simulink subsystem "InverseServoValveLinkage"  (R2020b)
settings: Solver=VariableStepAuto  StartTime=0.0  StopTime=10.0  RelTol=1e-3
model mask{servoValveSignConvention=ServoValveSignConvention.POSITIVE_AWAY_FROM_VALVE, valveCloseHandleRotationDirection=ValveCloseHandleRotationDirection.AWAY_FROM_SERVO, g=21, a=10.17, h=30.625, b=20.78, linkageServoAngleForClosedDegrees=217, servoCommandedCloseAngleDegrees=0}
  mask prompts: servoValveSignConvention "Servo valve sign convention"; valveCloseHandleRotationDirection "Valve handle close direction"; g "Distance between pivots (mm)"; a "Length of crank arm (mm)"; h "Length of coupler arm (mm)"; b "Length of rocket arm (mm)"; linkageServoAngleForClosedDegrees "Servo angle for closed valve degrees (in linkage angle convention)"; servoCommandedCloseAngleDegrees "Angle to command to servo for closed valve degrees"
undefined symbols (not defined in the file or in its folder): linkageValveAngleForOpenDegrees
settings Model: Creator=Edward  LastModifiedBy=Edward

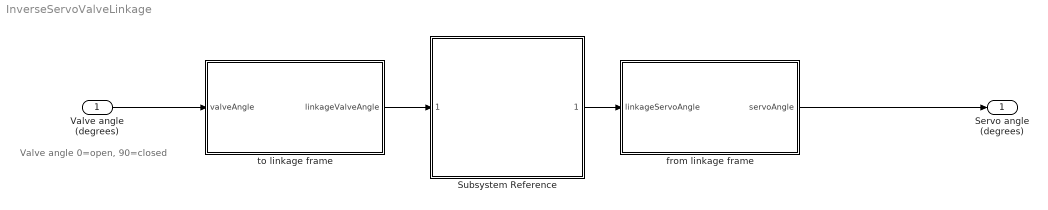
== system InverseServoValveLinkage ==
  note: Valve angle 0=open, 90=closed
  Valve angle (degrees) : Inport
  Subsystem Reference : Subsystem  ReferencedSubsystem=AnalyticInverseFourBarLinkage  g=g  a=a  h=h  b=b  solutionSelector=1
  from linkage frame : MATLAB Function  TreatAsAtomicUnit=on
  to linkage frame : MATLAB Function  TreatAsAtomicUnit=on
  Servo angle (degrees) : Outport
  wires:
  from linkage frame/1(servoAngle) -> Servo angle (degrees)/1
  Valve angle (degrees)/1 -> to linkage frame/1(valveAngle)
  Subsystem Reference/1 -> from linkage frame/1(linkageServoAngle)
  to linkage frame/1(linkageValveAngle) -> Subsystem Reference/1

== matlab function InverseServoValveLinkage/from linkage frame ==
  data: linkageServoAngle input; servoAngle output; linkageServoAngleForClosedDegrees parameter; servoCommandedCloseAngleDegrees parameter; servoValveSignConvention parameter Enum: ServoValveSignConvention; valveCloseHandleRotationDirection parameter Enum: ValveCloseHandleRotationDirection
function servoAngle = fcn(linkageServoAngle, linkageServoAngleForClosedDegrees, ...
servoCommandedCloseAngleDegrees, servoValveSignConvention, valveCloseHandleRotationDirection)
%Get actual servo angle from linkage coordinate system servoAngle
servoAngle = -1;
if(servoValveSignConvention == ServoValveSignConvention.POSITIVE_AWAY_FROM_VALVE)
    if(valveCloseHandleRotationDirection == ValveCloseHandleRotationDirection.TOWARDS_SERVO)
        servoAngle = clampDegreeAngle(linkageServoAngle-linkageServoAngleForClosedDegrees+servoCommandedCloseAngleDegrees);
    elseif(valveCloseHandleRotationDirection == ValveCloseHandleRotationDirection.AWAY_FROM_SERVO)
        servoAngle = clampDegreeAngle(-(linkageServoAngle-linkageServoAngleForClosedDegrees)+servoCommandedCloseAngleDegrees);
    end
elseif (servoValveSignConvention == ServoValveSignConvention.POSITIVE_TOWARDS_VALVE)
    if(valveCloseHandleRotationDirection == ValveCloseHandleRotationDirection.TOWARDS_SERVO)
        servoAngle = clampDegreeAngle(-(linkageServoAngle - servoCommandedCloseAngleDegrees) + linkageServoAngleForClosedDegrees);
    elseif(valveCloseHandleRotationDirection == ValveCloseHandleRotationDirection.AWAY_FROM_SERVO)
        servoAngle = clampDegreeAngle(linkageServoAngle-linkageServoAngleForClosedDegrees+servoCommandedCloseAngleDegrees);
    end
end
if(servoAngle >= 300)
   servoAngle = servoAngle-360; 
end

== matlab function InverseServoValveLinkage/to linkage frame ==
  data: valveAngle input; linkageValveAngle output; linkageValveAngleForOpenDegrees parameter; valveCloseHandleRotationDirection parameter Enum: ValveCloseHandleRotationDirection
function linkageValveAngle = fcn(valveAngle, linkageValveAngleForOpenDegrees, ...
    valveCloseHandleRotationDirection)
%Get actual valve angle (0=open,90=closed) from linkage coordinate system
linkageValveAngle = -1;
if(valveCloseHandleRotationDirection == ValveCloseHandleRotationDirection.TOWARDS_SERVO)
    linkageValveAngle = clampDegreeAngle(valveAngle+linkageValveAngleForOpenDegrees);
elseif(valveCloseHandleRotationDirection == ValveCloseHandleRotationDirection.AWAY_FROM_SERVO)
    linkageValveAngle = clampDegreeAngle(-valveAngle+linkageValveAngleForOpenDegrees);
end
